simulink model "es1_sim"  (Simulink 7.0)
settings: Solver=ode45  StartTime=0.0  StopTime=10  MaxStep=0.1  RelTol=1e-3  AbsTol=1e-3
values from neighbouring files (symbols this model uses):
  A = [-5 -11;4 7]    [es1a.m]    (also in es2a.m = [11 29;-5 -12])
  B = [1 1]'    [es1a.m]    (also in es2a.m)
  C = [1 0]    [es1a.m]    (also in es2a.m)
  G = [1 2;1 0]    [es1a.m]
  K = place(A,B,autoval)    [es2a.m]
  L = place(A',C',[-40 -50])'    [es2a.m]
undefined symbols (not defined in the file or in its folder): sigbuilder_block
settings Model: Creator=claudio  LastModifiedBy=claudio  ExtModeTrigMode=oneshot  ExtModeArmWhenConnect=off
settings DataIOCC: LimitDataPoints=off  SaveOutput=off  SaveTime=off
settings OptimizationCC: BooleanDataType=off  InlineInvariantSignals=on
settings DebuggingCC: SaveWithParameterizedLinksMsg=none  SignalResolutionControl=TryResolveAllWithWarning  SolverPrmCheckMsg=none  MultiTaskDSMMsg=warning  MultiTaskCondExecSysMsg=none  StrictBusMsg=None
settings HardwareCC: TargetUnknown=on
settings RTWCC: IncludeERTFirstTime=on
settings GRTTargetCC: TargetFcnLib=ansi_tfl_tmw.mat  ModelReferenceCompliant=off  MatFileLogging=off

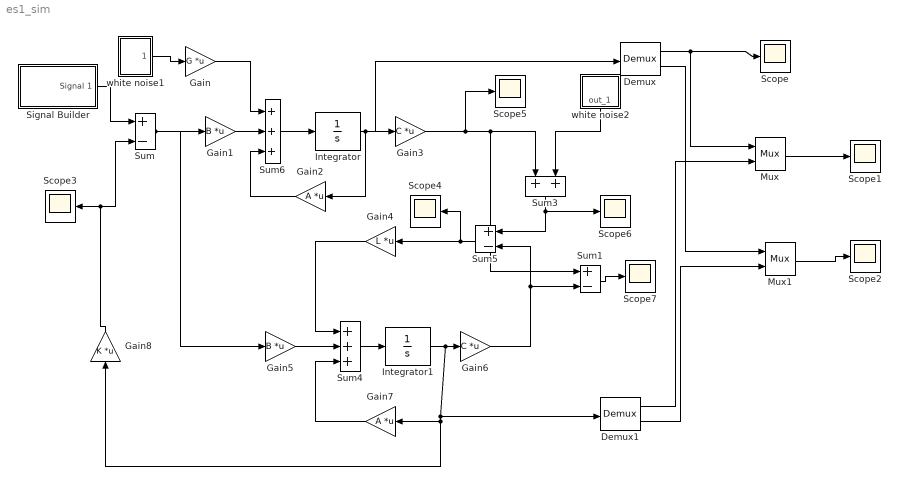
== system es1_sim ==
  Demux : Demux  Outputs=2
  Demux1 : Demux  Outputs=2
  Gain : Gain  Gain=G  Multiplication=Matrix(K*u)  ParameterDataType=sfix(16)  ParameterScaling=2^0  OutDataType=sfix(16)  OutScaling=2^0
  Gain1 : Gain  Gain=B  Multiplication=Matrix(K*u)  ParameterDataType=sfix(16)  ParameterScaling=2^0  OutDataType=sfix(16)  OutScaling=2^0
  Gain2 : Gain  Orientation=left  Gain=A  Multiplication=Matrix(K*u)  ParameterDataType=sfix(16)  ParameterScaling=2^0  OutDataType=sfix(16)  OutScaling=2^0
  Gain3 : Gain  Gain=C  Multiplication=Matrix(K*u)  ParameterDataType=sfix(16)  ParameterScaling=2^0  OutDataType=sfix(16)  OutScaling=2^0
  Gain4 : Gain  Orientation=left  Gain=L  Multiplication=Matrix(K*u)  ParameterDataType=sfix(16)  ParameterScaling=2^0  OutDataType=sfix(16)  OutScaling=2^0
  Gain5 : Gain  Gain=B  Multiplication=Matrix(K*u)  ParameterDataType=sfix(16)  ParameterScaling=2^0  OutDataType=sfix(16)  OutScaling=2^0
  Gain6 : Gain  Gain=C  Multiplication=Matrix(K*u)  ParameterDataType=sfix(16)  ParameterScaling=2^0  OutDataType=sfix(16)  OutScaling=2^0
  Gain7 : Gain  Orientation=left  Gain=A  Multiplication=Matrix(K*u)  ParameterDataType=sfix(16)  ParameterScaling=2^0  OutDataType=sfix(16)  OutScaling=2^0
  Gain8 : Gain  Orientation=up  Gain=K  Multiplication=Matrix(K*u)  ParameterDataType=sfix(16)  ParameterScaling=2^0  OutDataType=sfix(16)  OutScaling=2^0
  Integrator : Integrator  InitialCondition=[ 0 0 ]
  Integrator1 : Integrator  InitialCondition=[ 0 0 ]
  Mux : Mux  Inputs=2
  Mux1 : Mux  Inputs=2
  Scope{,1..7} (8 alike) : Scope
      Scope settings: TimeRange=10
      Scope2 settings: SaveName=ScopeData2
      Scope3 settings: SaveName=ScopeData3
      Scope4 settings: SaveName=ScopeData4
      Scope5 settings: TimeRange=10  SaveName=ScopeData5
      Scope6 settings: TimeRange=10  SaveName=ScopeData6
      Scope7 settings: TimeRange=10  SaveName=ScopeData7
  Signal Builder : Subsystem  Tag=STV Subsys  LoadFcn=sigbuilder_block('load',[403.5 179.25 550.5 362.25 ]);  StartFcn=sigbuilder_block('start');  StopFcn=sigbuilder_block('stop');  ClipboardFcn=sigbuilder_block('clipboard');  mask(Sigbuilder block){}
      mask help: Sigbuilder GUI
      mask init:
      | if ~strcmp(get_param(bdroot(gcbh),'SimulationStatus'),'stopped') tuvar = sigbuilder_block('maskInit'); end
      settings: CopyFcn=sigbuilder_block('copy');  DeleteFcn=sigbuilder_block('delete');  ModelCloseFcn=sigbuilder_block('modelClose');  PreSaveFcn=sigbuilder_block('preSave');  NameChangeFcn=sigbuilder_block('namechange');  OpenFcn=sigbuilder_block('open',[403.5 179.25 550.5 362.25 ]);  CloseFcn=sigbuilder_block('close');
      mask Display: plot(0,0,100,100,[10,10,40,40,10],[80,20,20,80,80],[40,10],[50,50], [40,27,10],[65,72,56],[40,25,25,10],[28,28,43,43]);
  Sum : Sum  Inputs=+-  OutDataType=sfix(16)  OutScaling=2^0  SaturateOnIntegerOverflow=on  InputSameDT=on
  Sum1 : Sum  Inputs=+-  OutDataType=sfix(16)  OutScaling=2^0  SaturateOnIntegerOverflow=on  InputSameDT=on
  Sum3 : Sum  Orientation=down  OutDataType=sfix(16)  OutScaling=2^0  SaturateOnIntegerOverflow=on  InputSameDT=on
  Sum4 : Sum  Inputs=+++  OutDataType=sfix(16)  OutScaling=2^0  SaturateOnIntegerOverflow=on  InputSameDT=on
  Sum5 : Sum  Orientation=left  Inputs=+-  OutDataType=sfix(16)  OutScaling=2^0  SaturateOnIntegerOverflow=on  InputSameDT=on
  Sum6 : Sum  Inputs=+++  OutDataType=sfix(16)  OutScaling=2^0  SaturateOnIntegerOverflow=on  InputSameDT=on
  white noise1 : Subsystem  mask(Continuous White Noise.){@1=Rw, @2=0.1, @3=12}
      mask prompts: @1 "Noise Variance:"; @2 "Sample Time:"; @3 "Seed"
      mask help:
      | White noise for continuous (s-domain) systems.
      | Band-limited using zero-order-hold.
      mask init:
      | Cov = @1; Ts = @2; seed = @3;
      mask Help: Implemented using white noise into Zero Order Hold block. For faster simulation set sample time to highest value possible but in accordance with the fastest dynamics of system.
      mask Display: plot(1:20,rand(1,20))
  white noise2 : Subsystem  Orientation=down  mask(Continuous White Noise.){@1=Rv, @2=0.1, @3=12}
      mask prompts: @1 "Noise Variance:"; @2 "Sample Time:"; @3 "Seed"
      mask help:
      | White noise for continuous (s-domain) systems.
      | Band-limited using zero-order-hold.
      mask init:
      | Cov = @1; Ts = @2; seed = @3;
      mask Help: Implemented using white noise into Zero Order Hold block. For faster simulation set sample time to highest value possible but in accordance with the fastest dynamics of system.
      mask Display: plot(1:20,rand(1,20))
  wires:
  Integrator1/1 -> Demux1/1, Gain7/1, Gain8/1, Gain6/1
  Sum4/1 -> Integrator1/1
  Gain7/1 -> Sum4/3
  Gain5/1 -> Sum4/2
  Gain3/1 -> Scope5/1, Sum3/1, Sum1/1
  Sum3/1 -> Sum5/1, Scope6/1
  Gain6/1 -> Sum5/2, Sum1/2
  Gain4/1 -> Sum4/1
  Integrator/1 -> Demux/1, Gain2/1, Gain3/1
  Sum5/1 -> Gain4/1, Scope4/1
  white noise2/1(out_1) -> Sum3/2
  Sum6/1 -> Integrator/1
  Gain8/1 -> Sum/2, Scope3/1
  Gain1/1 -> Sum6/2
  white noise1/1(out_1) -> Gain/1
  Gain/1 -> Sum6/1
  Gain2/1 -> Sum6/3
  Sum/1 -> Gain1/1, Gain5/1
  Demux1/1 -> Mux/2
  Demux/1 -> Mux/1, Scope/1
  Mux/1 -> Scope1/1
  Demux/2 -> Mux1/1
  Demux1/2 -> Mux1/2
  Mux1/1 -> Scope2/1
  Signal Builder/1(Signal 1) -> Sum/1
  Sum1/1 -> Scope7/1

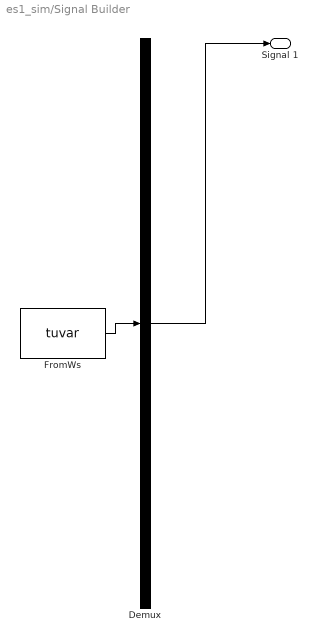
== system es1_sim/Signal Builder ==
  Demux : Demux  Tag=STV Demux  Outputs=1
  FromWs : FromWorkspace  Tag=STV FromWs  VariableName=tuvar  SampleTime=0  SigBuilderData=DataTag0  VnvData=DataTag1
      SigBuilderData=|
      | channels.label = 'Signal 1'
      | channels.allXData = {[0 3 3 4 4 10]}
      | channels.allYData = {[0 0 5 5 0 0]}
      | common.afterFinalStr = 'Extrapolate'
      | common.sampleTime = 0
      | dataSet.timeRange = [0 10]
      | dataSet.name = 'Group 1'
  Signal 1 : Outport  Tag=STV Outport  OutDataType=sfix(16)  OutScaling=2^0
  wires:
  Demux/1 -> Signal 1/1
  FromWs/1 -> Demux/1

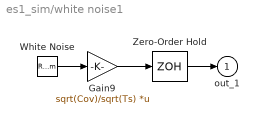
== system es1_sim/white noise1 ==
  Gain9 : Gain  Gain=sqrt(Cov)/sqrt(Ts)  Multiplication=Matrix(K*u)  ParameterDataType=sfix(16)  ParameterScaling=2^0  OutDataType=sfix(16)  OutScaling=2^0
  White Noise : RandomNumber  Mean=zeros(length(Cov),1)  Variance=ones(length(Cov),1)  Seed=seed
  Zero-Order Hold : ZeroOrderHold  SampleTime=Ts
  out_1 : Outport  OutDataType=sfix(16)  OutScaling=2^0
  wires:
  Zero-Order Hold/1 -> out_1/1
  White Noise/1 -> Gain9/1
  Gain9/1 -> Zero-Order Hold/1

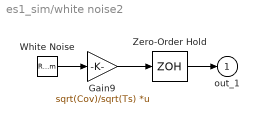
== system es1_sim/white noise2 ==
  Gain9 : Gain  Gain=sqrt(Cov)/sqrt(Ts)  Multiplication=Matrix(K*u)  ParameterDataType=sfix(16)  ParameterScaling=2^0  OutDataType=sfix(16)  OutScaling=2^0
  White Noise : RandomNumber  Mean=zeros(length(Cov),1)  Variance=ones(length(Cov),1)  Seed=seed
  Zero-Order Hold : ZeroOrderHold  SampleTime=Ts
  out_1 : Outport  OutDataType=sfix(16)  OutScaling=2^0
  wires:
  Gain9/1 -> Zero-Order Hold/1
  White Noise/1 -> Gain9/1
  Zero-Order Hold/1 -> out_1/1
